simulink subsystem "GyroStarTrackerReset"  (R2021a)
settings: Solver=VariableStepAuto  StartTime=0.0  StopTime=10.0  RelTol=1e-3
libraries: aerolibutil x1, sharedutil x1
settings Model: Creator=Laura  LastModifiedBy=Laura

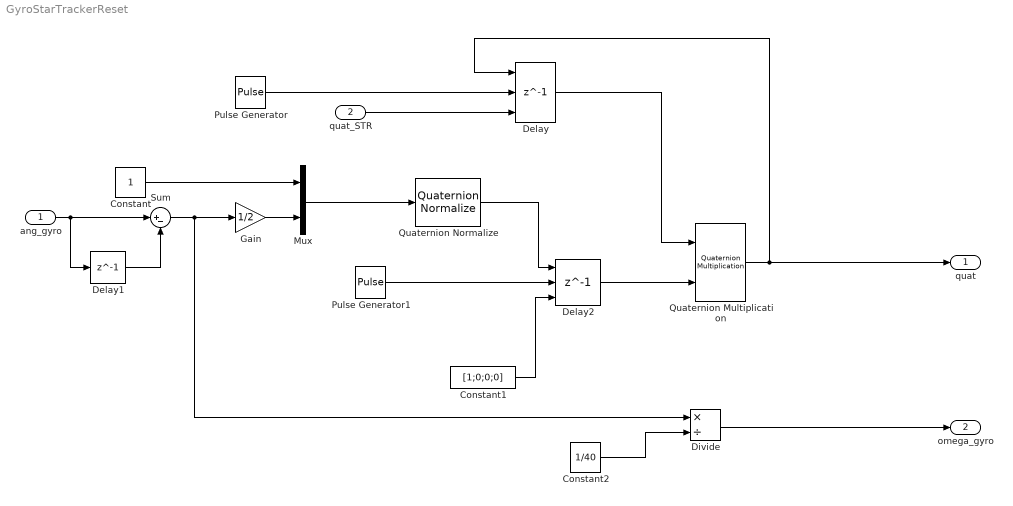
== system GyroStarTrackerReset ==
  ang_gyro : Inport  SampleTime=1/40
  quat_STR : Inport  Port=2  SampleTime=1/10
  Constant : Constant
  Constant1 : Constant  Value=[1;0;0;0]
  Constant2 : Constant  Value=1/40
  Delay : Delay  DelayLength=1  InitialConditionSource=Input port  ExternalReset=Rising
      settings: InputPortMap=u0,r5,p4
  Delay1 : Delay  DelayLength=1
  Delay2 : Delay  DelayLength=1  InitialConditionSource=Input port  ExternalReset=Rising
      settings: InputPortMap=u0,r5,p4
  Divide : Product  Inputs=*/
  Gain : Gain  Gain=1/2
  Mux : Mux  Inputs=2
  Pulse Generator : DiscretePulseGenerator  PulseType=Time based  Period=1/10  PulseWidth=5
  Pulse Generator1 : DiscretePulseGenerator  PulseType=Time based  Period=1/10  PulseWidth=5
  Quaternion Multiplication : aerolibutil/Quaternion Multiplication
  Quaternion Normalize : sharedutil/Quaternion Normalize  aMode=aMode
      settings: SourceProductBaseCode=AE,PW,DR,MT,UV,VE
  Sum : Sum  Inputs=|+-
  quat : Outport
  omega_gyro : Outport  Port=2
  wires:
  Divide/1 -> omega_gyro/1
  Constant2/1 -> Divide/2
  Gain/1 -> Mux/2
  Constant/1 -> Mux/1
  Mux/1 -> Quaternion Normalize/1
  Delay/1 -> Quaternion Multiplication/1
  Quaternion Multiplication/1 -> Delay/1, quat/1
  quat_STR/1 -> Delay/3
  Pulse Generator/1 -> Delay/2
  ang_gyro/1 -> Sum/1, Delay1/1
  Delay1/1 -> Sum/2
  Sum/1 -> Divide/1, Gain/1
  Delay2/1 -> Quaternion Multiplication/2
  Quaternion Normalize/1 -> Delay2/1
  Pulse Generator1/1 -> Delay2/2
  Constant1/1 -> Delay2/3
